simulink model "detector2"  (Simulink 2.20)
settings: Solver=FixedStepDiscrete  StartTime=0.0  StopTime=10.0  RelTol=1e-3  AbsTol=1e-6
undefined symbols (not defined in the file): firls
libraries: BufferedDSP x13, dspbuff x5, WinAudio x1
settings Model: SaveTime=off  SaveOutput=off  ConsistencyChecking=off  RTWPlaceOutputsASAP=off  RTWTemplateMakefile=e:\steve\matlab\simulink\grt_vc_sgm.tmf  RTWMakeCommand="make_rtw USER_SRCS=\"winmm.lib\" USER_INCLUDES=\"-Ie:\\steve\\matlab\\Simulink\\BufferedDSP\\src\\rtw\""

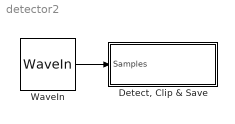
== system detector2 ==
  "Detect, Clip & Save" : Subsystem  mask(DetectClipNSave){buffersize=8192, f0=2000, f1=5000, threshold=2, numChannels=1, col_major=0, fs=22050}
      mask prompts: buffersize "Buffer Size:"; f0 "Lower Frequency (Hz):"; f1 "Upper Frequency (Hz):"; numChannels "Number of Channels:"; col_major "Column major channel order:"; fs "Sample Rate (Hz):"
      mask help: Detects acoustic events in a frequency band, clips, and saves them to disk.
      mask Help: Detects acoustic events in a frequency band, clips, and saves them to disk.
  WaveIn : WinAudio/WaveIn  sampleRateLit=22050  sampleWidthLit=16  stereo=off  col_major=1  buffersize=8192  bufTime=12
  wires:
  WaveIn/1 -> "Detect, Clip & Save"/1(Samples)

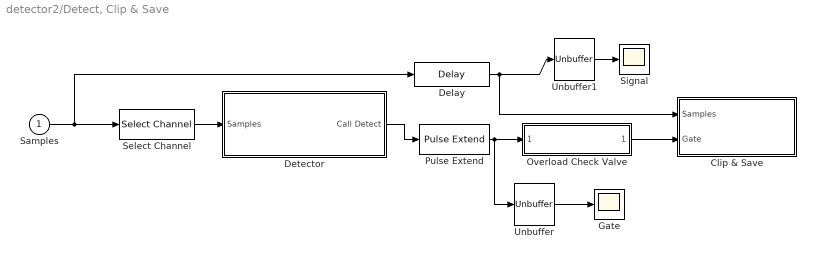
== system detector2/Detect, Clip & Save ==
  Samples : Inport  Port=1  PortWidth=buffersize * numChannels  SampleTime=-1
  Clip & Save : Subsystem  mask(ClipAndSave){buffersize=buffersize, fifosize=buffersize * 4, numChannels=numChannels, col_major=col_major, ftype=Wave, saveDir=c:\temp\calls, fname=Call, fnamestyle=Local time, fs=fs}
      mask prompts: buffersize "Buffer size (samples):"; fifosize "FIFO size (samples):"; numChannels "Number of Channels:"; col_major "Column major channel order"; ftype "File type:"; saveDir "Save Directory:"; fname "File Name Prefix:"; fnamestyle "File name time stamp:"; fs "Sample Rate (Hz):"
      mask help: Clips sections from "Samples" according to "Gate" and saves to Save Directory using File Name Prefix and adding a time stamp.
      mask Help: Clips sections from "Samples" according to "Gate" and saves to Save Directory using File Name Prefix and adding a time stamp.
      mask StyleString: edit,edit,edit,edit,popup(Wave|Mac Binary|Matlab|ASCII Float|ASCII Fixed|Binary Float|Binary Fixed|AIFF),edit,edit,popup(GMT|Local time|Time from start),edit
  Delay : BufferedDSP/Memory/Delay  buffersize=buffersize  delay=100  numChannels=numChannels  col_major=col_major
  Detector : Subsystem  mask(Detector){buffersize=buffersize, f0=f0, f1=f1, filterLength=100, threshold=threshold, numChannels=1, col_major=col_major, fs=fs}
      mask prompts: buffersize "Buffer Size:"; f0 "Lower Frequency (Hz):"; f1 "Upper Frequency (Hz):"; filterLength "Filter Length:"; numChannels "Number of Channels:"; col_major "Column major channel order:"; fs "Sample Rate:"
      mask help: Examines band-limited energy for events.
  Gate : Scope
      settings: TickLabels=on  TimeRange=auto  YMin=0  YMax=2  SaveToWorkspace=off  SaveName=ScopeData  LimitMaxRows=off  Decimation=100  SampleTime=1
  Overload Check Valve : Subsystem  mask(Overload Check Valve){buffersize=buffersize, guardTime=20, numEvents=40, fs=fs}
      mask prompts: buffersize "Buffer size (samples):"; guardTime "Length of time to check: (sec)"; numEvents "Prohibited number of events:"; fs "Sample rate (Hz):"
      mask help: Input and output signals are single channel Boolean event markers. If more than a prohibited number of events occur in a specified time duration, the output is zero. Otherwise, the input is passed through (ANDed) to the output.
      mask Help: Input and output signals are single channel Boolean event markers.  If more than a prohibited number of events occur in a specified time duration, the output is zero.  Otherwise, the input is passed through (ANDed) to the output.
      mask Display: disp(sprintf('%d events in %d sec',numEvents,guardTime))
  Pulse Extend : BufferedDSP/Pulse Shapers/Pulse Extend  buffersize=buffersize  lag=200  numChannels=1  col_major=col_major
  Select Channel : BufferedDSP/Multichannel/Select Channel  buffersize=buffersize  selectChannel=1  numChannels=numChannels  col_major=col_major
  Signal : Scope
      settings: TickLabels=on  TimeRange=auto  YMin=-1  YMax=1  SaveToWorkspace=off  SaveName=audio_signal  LimitMaxRows=off  Decimation=100  SampleTime=1
  Unbuffer : dspbuff/Unbuffer  num_chans=1  Ts=buffersize / fs
  Unbuffer1 : dspbuff/Unbuffer  num_chans=1  Ts=buffersize / fs
  wires:
  Detector/1(Call Detect) -> Pulse Extend/1
  Samples/1 -> Delay/1, Select Channel/1
  Unbuffer/1 -> Gate/1
  Select Channel/1 -> Detector/1(Samples)
  Unbuffer1/1 -> Signal/1
  Delay/1 -> Clip & Save/1(Samples), Unbuffer1/1
  Pulse Extend/1 -> Unbuffer/1, Overload Check Valve/1("      ")
  Overload Check Valve/1("     ") -> Clip & Save/2(Gate)

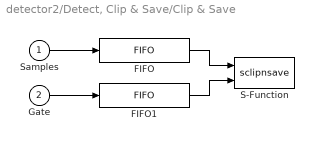
== system detector2/Detect, Clip & Save/Clip & Save ==
  Samples : Inport  Port=1  PortWidth=buffersize * numChannels  SampleTime=-1
  Gate : Inport  Port=2  PortWidth=buffersize  SampleTime=-1
  FIFO : BufferedDSP/Memory/FIFO  input_width=buffersize  output_width=fifosize  numChannels=numChannels  col_major=col_major
  FIFO1 : BufferedDSP/Memory/FIFO  input_width=buffersize  output_width=fifosize  numChannels=1  col_major=col_major
  S-Function : S-Function  FunctionName=sclipnsave  Parameters=buffersize fifosize numChannels col_major fname saveDir ftype fnamestyle fs  PortCounts=[]  SFunctionModules=''
  wires:
  FIFO1/1 -> S-Function/2
  FIFO/1 -> S-Function/1
  Gate/1 -> FIFO1/1
  Samples/1 -> FIFO/1

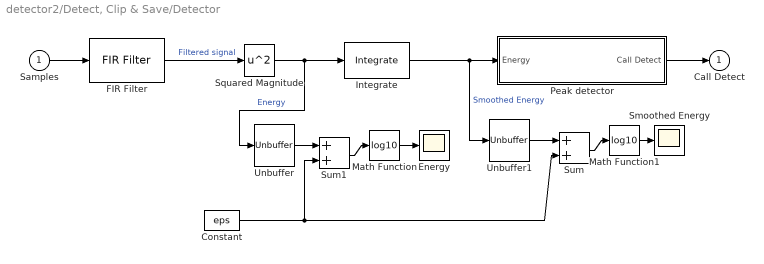
== system detector2/Detect, Clip & Save/Detector ==
  Samples : Inport  Port=1  PortWidth=buffersize *numChannels  SampleTime=-1
  Constant : Constant  Value=eps
  Energy : Scope
      settings: TickLabels=on  TimeRange=auto  YMin=-10  YMax=10  SaveToWorkspace=off  SaveName=ScopeData  LimitMaxRows=off  Decimation=100
  FIR Filter : BufferedDSP/Filter/Row Major/FIR Filter  input_width=buffersize  nfft_in=2*buffersize  h=firls(filterLength-1,[0 f0-100 f0 f1 f1+100 fs/2]/(fs/2),[0,0,1,1,0,0])  numChannels=numChannels
  Integrate : BufferedDSP/Filter/Integrate  buffersize=buffersize  integration_time=600  normalize=on  initial_value=0  numChannels=numChannels  col_major=col_major
  Math Function : Math  Operator=log10
  Math Function1 : Math  Operator=log10
  Peak detector : Subsystem  mask(PeakDetector){threshold=threshold, buffersize=buffersize, numChannels=numChannels, col_major=col_major, fs=fs}
      mask prompts: buffersize "Buffer Size:"; numChannels "Number of Channels:"; col_major "Column major channel order:"; fs "Sample Rate:"
      mask help: Finds large plateaus in an energy signal.
      mask Help: Finds large plateaus in an energy signal.
  Smoothed Energy : Scope
      settings: TickLabels=on  TimeRange=auto  YMin=-10  YMax=10  SaveToWorkspace=off  SaveName=ScopeData  LimitMaxRows=off  Decimation=100
  Squared Magnitude : Math  Operator=square
  Sum : Sum  Inputs=++
  Sum1 : Sum  Inputs=++
  Unbuffer : dspbuff/Unbuffer  num_chans=1  Ts=buffersize / fs
  Unbuffer1 : dspbuff/Unbuffer  num_chans=1  Ts=buffersize / fs
  Call Detect : Outport  Port=1  InitialOutput=0
  wires:
  Squared Magnitude/1 -> Unbuffer/1, Integrate/1  "Energy"
  Integrate/1 -> Unbuffer1/1, Peak detector/1(Energy)  "Smoothed Energy"
  Constant/1 -> Sum/2, Sum1/2
  Sum1/1 -> Math Function/1
  Unbuffer/1 -> Sum1/1
  Sum/1 -> Math Function1/1
  Unbuffer1/1 -> Sum/1
  Math Function1/1 -> Smoothed Energy/1
  Math Function/1 -> Energy/1
  FIR Filter/1 -> Squared Magnitude/1  "Filtered signal"
  Samples/1 -> FIR Filter/1
  Peak detector/1(Call Detect) -> Call Detect/1

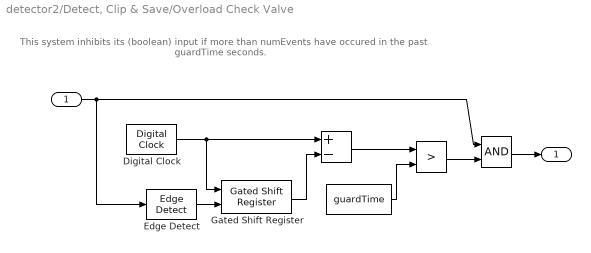
== system detector2/Detect, Clip & Save/Overload Check Valve ==
  note: This system inhibits its (boolean) input if
      | more than numEvents have occured
      | in the past guardTime seconds.
  "      " : Inport  Port=1  PortWidth=buffersize  SampleTime=-1
  " " : Constant  Value=guardTime
  "  " : RelationalOperator  Operator=>
  "    " : Logic  Operator=AND  Inputs=2
  "        " : Sum  Inputs=+-
  Digital Clock : BufferedDSP/Counters/Digital Clock  buffersize=buffersize  t0=guardTime+1  fs=fs
  Edge Detect : BufferedDSP/Pulse Shapers/Edge Detect  buffersize=buffersize  numChannels=1  col_major=1
  Gated Shift Register : BufferedDSP/Memory/Gated Shift Register  buffersize=buffersize  reg_size=numEvents  numChannels=1  col_major=1
  "     " : Outport  Port=1  InitialOutput=0
  wires:
  Digital Clock/1 -> Gated Shift Register/1, "        "/1
  Edge Detect/1 -> Gated Shift Register/2
  Gated Shift Register/1 -> "        "/2
  "        "/1 -> "  "/1
  " "/1 -> "  "/2
  "      "/1 -> "    "/1, Edge Detect/1
  "    "/1 -> "     "/1
  "  "/1 -> "    "/2

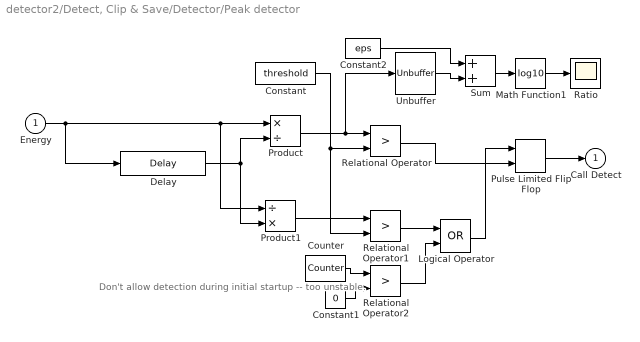
== system detector2/Detect, Clip & Save/Detector/Peak detector ==
  note: Don't allow detection during
      | initial startup -- too unstable.
  Energy : Inport  Port=1  PortWidth=buffersize * numChannels  SampleTime=-1
  Constant : Constant  Value=threshold
  Constant1 : Constant  Value=0
  Constant2 : Constant  Value=eps
  Counter : BufferedDSP/Counters/Counter  buffersize=buffersize  initial_count=1.2*buffersize  count_direction=Down  has_stop_count=on  stop_count=0  numChannels=numChannels  col_major=1  ts=-1
  Delay : BufferedDSP/Memory/Delay  buffersize=buffersize  delay=fix(fs * .020)  numChannels=numChannels  col_major=col_major
  Logical Operator : Logic  Operator=OR  Inputs=2
  Math Function1 : Math  Operator=log10
  Product : Product  Inputs=*/
  Product1 : Product  Inputs=/*
  Pulse Limited Flip Flop : BufferedDSP/Memory/Pulse Limited Flip Flop  buffersize=buffersize  initial_state=0  minLimit=fix(0.1 * fs)  maxLimit=fix(0.4 * fs)  numChannels=numChannels  col_major=col_major
  Ratio : Scope
      settings: TickLabels=on  TimeRange=auto  YMin=-1  YMax=1  SaveToWorkspace=off  SaveName=ScopeData  LimitMaxRows=off  Decimation=100  SampleTime=1
  Relational Operator : RelationalOperator  Operator=>
  Relational Operator1 : RelationalOperator  Operator=>
  Relational Operator2 : RelationalOperator  Operator=>
  Sum : Sum  Inputs=++
  Unbuffer : dspbuff/Unbuffer  num_chans=1  Ts=buffersize / fs
  Call Detect : Outport  Port=1  InitialOutput=0
  wires:
  Constant2/1 -> Sum/1
  Unbuffer/1 -> Sum/2
  Sum/1 -> Math Function1/1
  Math Function1/1 -> Ratio/1
  Relational Operator2/1 -> Logical Operator/2
  Constant1/1 -> Relational Operator2/2
  Counter/1 -> Relational Operator2/1
  Relational Operator1/1 -> Logical Operator/1
  Delay/1 -> Product1/2, Product/2
  Energy/1 -> Delay/1, Product/1, Product1/1
  Constant/1 -> Relational Operator/2, Relational Operator1/2
  Product1/1 -> Relational Operator1/1
  Product/1 -> Relational Operator/1, Unbuffer/1
  Pulse Limited Flip Flop/1 -> Call Detect/1
  Relational Operator/1 -> Pulse Limited Flip Flop/2
  Logical Operator/1 -> Pulse Limited Flip Flop/1
